simulink model "BPM_Dyno_harm_fmu"  (R2022b)
settings: configuration reference "ModelConfig_var" (kept outside this file)
InitFcn:
  | %% BUS initialization
  | Xabc.A = 0;
  | Xabc.B = 0;
  | Xabc.C = 0;
  | % -------------------------------------------------------------------------
  | Simulink.Bus.createObject(Xabc)
  | XabcBus = slBus1;
  | clear slBus1
  | 
  | %% Parameter Structure initialization
  | %Motor_prm_init_bpm;
model workspace (MAT data in the model file):
  Mech_HAs_CF = 0
  Mech_HAs_J_drum = 0
  Mech_HAs_TR = 0
  Mech_HAs_damp = 0
  Mech_HAs_m_unb = 0
  Mech_HAs_r_unb = 0
  Mech_VAa_J_basket = 0
  Mech_VAa_J_impeller = 0
  Mech_VAa_basket_dens = 0
  Mech_VAa_basket_dia = 0
  Mech_VAa_belt_ratio = 0
  Mech_VAa_clothes_mass = 0
  Mech_VAa_gear_ratio = 0
  Mech_VAa_imp_dens = 0
  Mech_VAa_water_vol = 0
  Mech_VAs_D_r = 0
  Mech_VAs_I_zt = 0
  Mech_VAs_K = 2700
  Mech_VAs_T_f = 0
  Mech_VAs_belt_rat = 0
  Mech_VAs_d = 0
  Mech_VAs_e = 0
  Mech_VAs_m_b1 = 0
  Mech_VAs_m_b2 = 0
  Mech_VAs_m_d = 0
  Mech_VAs_m_t = 0
  Mech_VAs_m_u = 0
  Time_step = 0.0001
  Time_step_solver = 0
  bpm_B = 0
  bpm_Ipk = [0 1 2 3 4 5 6 7]
  bpm_Jrotor = 0
  bpm_Ld_0 = 0.02117
  bpm_Ld_a = [0.02117 0.02117 0.02117 0.02117 0.02117 0.02117 0.02117 0.02117]
  bpm_Loss_Power = [0 1 2 3 4 5 6 7]
  bpm_Loss_Speed = [0 1 2 3 4 5 6 7]
  bpm_Loss_flag = 1
  bpm_Loss_th = 10
  bpm_Lq_0 = 0.02117
  bpm_Lq_b = [0.02117 0.02117 0.02117 0.02117 0.02117 0.02117 0.02117 0.02117]
  bpm_Ls_sat_flag = 1
  bpm_NPP = 0
  bpm_PM_flux_h1_0 = 0
  bpm_PM_rotor_alpha = 0
  bpm_Rs_0 = 0
  bpm_Rs_stator_alpha = 0
  bpm_Rsa_aux = 0
  bpm_Rsb_aux = 0
  bpm_Rsc_aux = 0
  bpm_TR = 1
  bpm_Temp_rotor_0 = 0
  bpm_Temp_stator_0 = 0
undefined symbols (not defined in the file): Motor, TimeSteps
settings Model: Creator=BEDNASA  LastModifiedBy=BEATOA
settings ConfigSetRef: SourceName=ModelConfig_var  SourceLocation=Base Workspace

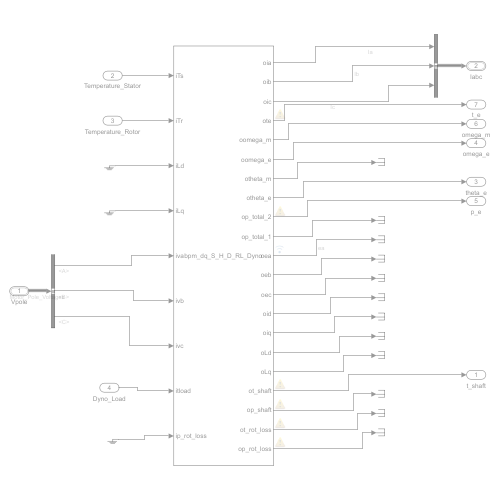
[thumbnail: Simulink's stored preview of the top-level diagram]
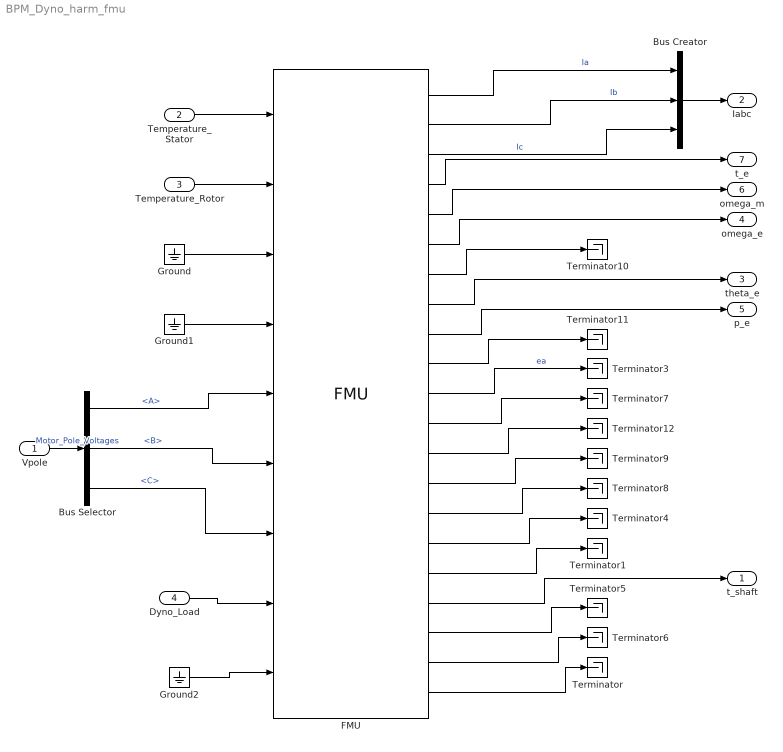
== system BPM_Dyno_harm_fmu ==
  Vpole : Inport  OutDataTypeStr=Bus: XabcBus
  Temperature_Stator : Inport  Port=2
  Temperature_Rotor : Inport  Port=3
  Dyno_Load : Inport  Port=4
  Bus Creator : BusCreator  Inputs=3
  Bus Selector : BusSelector  OutputSignals=A,B,C
  FMU : FMU  FMUName=bpm_dq_S_H_D_RL_Dyno.fmu  FMUMode=CoSimulation  Rs0=Motor.Electrical.Rs_a_Ref  Rs_a0=Motor.Electrical.Rs_a_Ref  Rs_b0=Motor.Electrical.Rs_b_Ref  Rs_c0=Motor.Electrical.Rs_c_Ref  phiPM1=Motor.Electrical.PM_Flux_f01  NPP=Motor.Electrical.p_Pole_Pairs  Jrotor=Motor.Mechanical.Jrotor  B=Motor.Mechanical.B  Ts=TimeSteps.ModelStep  TsRef=22  TrRef=22  alpha_s=0.004  d_magnet=0.00206  flux_harm_enable=1  phiPM2=Motor.Electrical.PM_Flux_f02  phiPM3=Motor.Electrical.PM_Flux_f03  phiPM4=Motor.Electrical.PM_Flux_f04  phiPM5=Motor.Electrical.PM_Flux_f05  phiPM6=Motor.Electrical.PM_Flux_f06  phiPM7=Motor.Electrical.PM_Flux_f07  phiPM8=Motor.Electrical.PM_Flux_f08  phiPM9=Motor.Electrical.PM_Flux_f09  phiPM10=Motor.Electrical.PM_Flux_f10  phiPM11=Motor.Electrical.PM_Flux_f11  phiPM12=Motor.Electrical.PM_Flux_f12  phiPM13=Motor.Electrical.PM_Flux_f13  Ls_sat_input_flag=int32(1)  I_pk0=Motor.Inductance_Variation.I_pk0  I_pk1=Motor.Inductance_Variation.I_pk1  I_pk2=Motor.Inductance_Variation.I_pk2  I_pk3=Motor.Inductance_Variation.I_pk3  I_pk4=Motor.Inductance_Variation.I_pk4  I_pk5=Motor.Inductance_Variation.I_pk5  I_pk6=Motor.Inductance_Variation.I_pk6  I_pk7=Motor.Inductance_Variation.I_pk7  Ld_a0=Motor.Inductance_Variation.Ld_a0  Ld_a1=Motor.Inductance_Variation.Ld_a1  Ld_a2=Motor.Inductance_Variation.Ld_a2  Ld_a3=Motor.Inductance_Variation.Ld_a3  Ld_a4=Motor.Inductance_Variation.Ld_a4  Ld_a5=Motor.Inductance_Variation.Ld_a5  Ld_a6=Motor.Inductance_Variation.Ld_a6  Ld_a7=Motor.Inductance_Variation.Ld_a7  Lq_b0=Motor.Inductance_Variation.Lq_b0  Lq_b1=Motor.Inductance_Variation.Lq_b1  Lq_b2=Motor.Inductance_Variation.Lq_b2  Lq_b3=Motor.Inductance_Variation.Lq_b3  Lq_b4=Motor.Inductance_Variation.Lq_b4  Lq_b5=Motor.Inductance_Variation.Lq_b5  Lq_b6=Motor.Inductance_Variation.Lq_b6  Lq_b7=Motor.Inductance_Variation.Lq_b7  Rot_Loss_input_flag=int32(1)  Rot_Loss_enable=1  Rot_Loss_omega_th=5  Rot_Loss_Speed0=Motor.Power_Loss.Rot_Loss_Speed0  Rot_Loss_Speed1=Motor.Power_Loss.Rot_Loss_Speed1+0.1  Rot_Loss_Speed2=Motor.Power_Loss.Rot_Loss_Speed2+0.2  Rot_Loss_Speed3=Motor.Power_Loss.Rot_Loss_Speed3+0.3  Rot_Loss_Speed4=Motor.Power_Loss.Rot_Loss_Speed4+0.4  Rot_Loss_Speed5=Motor.Power_Loss.Rot_Loss_Speed5+0.5  Rot_Loss_Speed6=Motor.Power_Loss.Rot_Loss_Speed6+0.6  Rot_Loss_Speed7=Motor.Power_Loss.Rot_Loss_Speed7+0.7  Rot_Loss_Power0=Motor.Power_Loss.Rot_Loss_Power0  Rot_Loss_Power1=Motor.Power_Loss.Rot_Loss_Power1  Rot_Loss_Power2=Motor.Power_Loss.Rot_Loss_Power2  Rot_Loss_Power3=Motor.Power_Loss.Rot_Loss_Power3  Rot_Loss_Power4=Motor.Power_Loss.Rot_Loss_Power4  Rot_Loss_Power5=Motor.Power_Loss.Rot_Loss_Power5  Rot_Loss_Power6=Motor.Power_Loss.Rot_Loss_Power6  Rot_Loss_Power7=Motor.Power_Loss.Rot_Loss_Power7  mask(bpm_dq_S_H_D_RL_Dyno [Co-Simulation, v2.0]){}
      mask Display:
      | disp('bpm_dq_S_H_D_RL_Dyno');
      | port_label('output',1,'oia');
      | port_label('output',2,'oib');
      | port_label('output',3,'oic');
      | port_label('output',4,'ote');
      | port_label('output',5,'oomega_m');
      | port_label('output',6,'oomega_e');
      | port_label('output',7,'otheta_m');
      | port_label('output',8,'otheta_e');
      | port_label('output',9,'op_total_2');
      | port_label('output',10,'op_total_1');
      | port_label('output',11,'oea');
      | port_label('output',12,'oeb');
      | port_label('output',13,'oec');
      | port_label('output',14,'oid');
      | port_label('output',15,'oiq');
      | port_label('output',16,'oLd');
      | port_label('output',17,'oLq');
      | port_label('output',18,'ot_shaft');
      | port_label('output',19,'op_shaft');
      | port_label('output',20,'ot_rot_loss');
      | port_label('output',21,'op_rot_loss');
      | port_label('input',1,'iTs');
      | port_label('input',2,'iTr');
      | port_label('input',3,'iLd');
      | port_label('input',4,'iLq');
      | port_label('input',5,'iva');
      | port_label('input',6,'ivb');
      | port_label('input',7,'ivc');
      | port_label('input',8,'itload');
      | port_label('input',9,'ip_rot_loss');
  Ground : Ground
  Ground1 : Ground
  Ground2 : Ground
  Terminator{,1,3..12} (12 alike) : Terminator
  t_shaft : Outport  VectorParamsAs1DForOutWhenUnconnected=off
  Iabc : Outport  Port=2  OutDataTypeStr=Bus: XabcBus  VectorParamsAs1DForOutWhenUnconnected=off
  theta_e : Outport  Port=3  VectorParamsAs1DForOutWhenUnconnected=off
  omega_e : Outport  Port=4  VectorParamsAs1DForOutWhenUnconnected=off
  p_e : Outport  Port=5  VectorParamsAs1DForOutWhenUnconnected=off
  omega_m : Outport  Port=6  VectorParamsAs1DForOutWhenUnconnected=off
  t_e : Outport  Port=7  VectorParamsAs1DForOutWhenUnconnected=off
  wires:
  FMU/21 -> Terminator/1
  FMU/17 -> Terminator1/1
  FMU/11 -> Terminator3/1  "ea"
  FMU/16 -> Terminator4/1
  FMU/5 -> omega_m/1
  FMU/6 -> omega_e/1
  FMU/8 -> theta_e/1
  FMU/4 -> t_e/1
  FMU/18 -> t_shaft/1
  FMU/19 -> Terminator5/1
  FMU/20 -> Terminator6/1
  FMU/12 -> Terminator7/1
  FMU/9 -> p_e/1
  FMU/15 -> Terminator8/1
  FMU/7 -> Terminator10/1
  FMU/10 -> Terminator11/1
  Bus Selector/3 -> FMU/7  "<C>"
  Bus Selector/2 -> FMU/6  "<B>"
  Vpole/1 -> Bus Selector/1  "Motor_Pole_Voltages"
  FMU/2 -> Bus Creator/2  "Ib"
  Bus Creator/1 -> Iabc/1
  FMU/1 -> Bus Creator/1  "Ia"
  FMU/3 -> Bus Creator/3  "Ic"
  Bus Selector/1 -> FMU/5  "<A>"
  FMU/13 -> Terminator12/1
  FMU/14 -> Terminator9/1
  Temperature_Rotor/1 -> FMU/2
  Temperature_Stator/1 -> FMU/1
  Ground/1 -> FMU/3
  Ground1/1 -> FMU/4
  Dyno_Load/1 -> FMU/8
  Ground2/1 -> FMU/9
